simulink model "steeringwheel"  (R2018b)
settings: Solver=ode45  StartTime=0.0  StopTime=10  MaxStep=1e-2  RelTol=1e-6
settings Model: Creator=jinwooro  LastModifiedBy=jinwooro

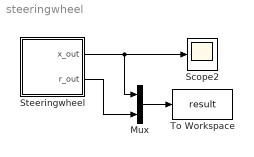
== system steeringwheel ==
  Mux : Mux  Inputs=2
  Scope2 : Scope
  Steeringwheel : Stateflow chart  TreatAsAtomicUnit=on
  To Workspace : ToWorkspace  VariableName=result  SaveFormat=Timeseries  SampleTime=-1
  wires:
  Steeringwheel/1(x_out) -> Mux/1, Scope2/1
  Mux/1 -> To Workspace/1
  Steeringwheel/2(r_out) -> Mux/2

== stateflow chart steeringwheel/Steeringwheel ==
  settings: updateMethod=CONTINUOUS
  state LeftTurn
    du:
    r_dot = 1;
    r_out = r;
    x_out = cos(r);
  state RightTurn
    du:
    r_dot = -3*pi;
    r_out = r;
    x_out = cos(r);
  (default) -> LeftTurn : {r = 0;}
  LeftTurn -> RightTurn : [cos(r) <= -0.99]
  RightTurn -> LeftTurn : [cos(r) >= 0.99]
  data: r local; x_out output; r_out output
  data r settings: updateMethod=SF_CONTINUOUS_TIME_DATA
